simulink model "PenduloSimpleControlDifuso"  (R2018a)
settings: Solver=VariableStepAuto  StartTime=0.0  StopTime=100  FixedStep=0.01  RelTol=1e-3
values from neighbouring files (symbols this model uses):
  g = -1    [D_particiones_a_h.m]    (also in InterpolacionHERMITE.m = 1)
  k = k+1    (= 2)    [EulerHEUN.m]    (also in GraficaImplicita.m; HeunFunc.m; IntegralesDefinidas.m = subs(vecSol(ii),y); InterpolacionHERMITE.m = 1)
  l = (l+1)    (= 2)    [CuadrosMAGICOS.m]    (also in LangrangeF.m = l*((vfx-x(j+1))/(x(i+1)-x(j+1))); Matrix.m = length(A))
  m = 1    [CuadrosMAGICOS.m]    (also in ExperimentoInstrumentaacion.m = (N*sxy-sx*sy)/(N*sxx-sx*sx); InterpolationNewton.m = 2; Jose.m = 2; JoseCarlos.m)
undefined symbols (not defined in the file or in its folder): K1, K2, L1, L2
settings Model: Creator=Benjamin Nicolas  LastModifiedBy=Benjamin Nicolas

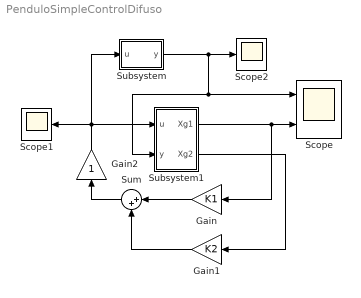
== system PenduloSimpleControlDifuso ==
  Gain : Gain  Gain=K1
  Gain1 : Gain  Gain=K2
  Gain2 : Gain
  Scope : Scope  NumInputPorts=2
  Scope1 : Scope
  Scope2 : Scope
  Subsystem : Subsystem
  Subsystem1 : Subsystem
  Sum : Sum  Inputs=|++
  wires:
  Subsystem/1(y) -> Scope2/1, Scope/1, Subsystem1/2(y)
  Gain/1 -> Sum/1
  Gain1/1 -> Sum/2
  Subsystem1/1(Xg1) -> Scope/2, Gain/1
  Subsystem1/2(Xg2) -> Gain1/1
  Sum/1 -> Gain2/1
  Gain2/1 -> Scope1/1, Subsystem1/1(u), Subsystem/1(u)

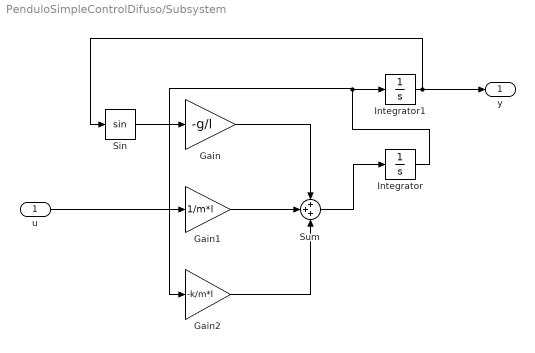
== system PenduloSimpleControlDifuso/Subsystem ==
  u : Inport
  Gain : Gain  Gain=-g/l
  Gain1 : Gain  Gain=1/m*l
  Gain2 : Gain  Gain=-k/m*l
  Integrator : Integrator  InitialCondition=0.5
  Integrator1 : Integrator  InitialCondition=0.5
  Sin : Trigonometry
  Sum : Sum  Inputs=+++
  y : Outport
  wires:
  Gain/1 -> Sum/1
  Gain1/1 -> Sum/2
  u/1 -> Gain1/1
  Sum/1 -> Integrator/1
  Integrator1/1 -> y/1, Sin/1
  Sin/1 -> Gain/1
  Gain2/1 -> Sum/3
  Integrator/1 -> Integrator1/1, Gain2/1

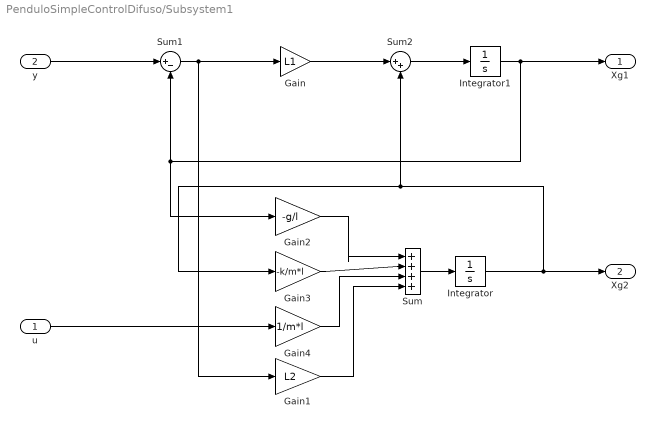
== system PenduloSimpleControlDifuso/Subsystem1 ==
  u : Inport
  y : Inport  Port=2
  Gain : Gain  Gain=L1
  Gain1 : Gain  Gain=L2
  Gain2 : Gain  Gain=-g/l
  Gain3 : Gain  Gain=-k/m*l
  Gain4 : Gain  Gain=1/m*l
  Integrator : Integrator  InitialCondition=0.5
  Integrator1 : Integrator  InitialCondition=pi/2
  Sum : Sum  Inputs=|++++
  Sum1 : Sum  Inputs=|+-
  Sum2 : Sum  Inputs=|++
  Xg1 : Outport
  Xg2 : Outport  Port=2
  wires:
  Integrator/1 -> Sum2/2, Gain3/1, Xg2/1
  Sum/1 -> Integrator/1
  Gain2/1 -> Sum/1
  Gain3/1 -> Sum/2
  Sum2/1 -> Integrator1/1
  Integrator1/1 -> Xg1/1, Sum1/2, Gain2/1
  Gain/1 -> Sum2/1
  Gain4/1 -> Sum/3
  y/1 -> Sum1/1
  Gain1/1 -> Sum/4
  Sum1/1 -> Gain/1, Gain1/1
  u/1 -> Gain4/1
